simulink model "ASM_Traffic_V2X_Complete_Model_2"  (R2019a)
settings: Solver=ode1  StartTime=SIM.tstart.v  StopTime=Inf  FixedStep=SIM.StepSize.v  RelTol=1e-3
PostLoadFcn:
  | if any(exist('dsrtsu_mdlpostloadfcn', 'file') ~= 0), dsrtsu_mdlpostloadfcn('Execute', bdroot); end
  | try, asm_mdl_postloadfcn(bdroot, 'UpdateModel', 2200); catch, disp(lasterr); end,
undefined symbols (not defined in the file): _SensorPnts_1, _SensorPnts_13, _SensorPnts_17, _SensorPnts_21, _SensorPnts_25, _SensorPnts_29, _SensorPnts_33, _SensorPnts_37, _SensorPnts_41, _SensorPnts_45, _SensorPnts_49, _SensorPnts_5, _SensorPnts_53, _SensorPnts_57, _SensorPnts_9, _to_, CPT, G5A, ITS, MDL, rad, s_to_rpm, SIM
libraries: simulink x169, ASM_VehicleDynamics_lib x126, ASM_Traffic_lib x83, ASM_Utils_lib x49, mdbs x45, ASM_Environment_lib x17, dspindex x12, dsaV2xLibraryAux x10, dsmpblib x6, dsaV2xAsn1Library x4, dsaV2xLibrary x4, ASM_BrakeHydraulics_lib x4
(part 5 of 36)

== system ASM_Traffic_V2X_Complete_Model_2/MDL/SoftECU/Soft_ECU_Engine_Basic ==
  n_Engine[rpm] : Inport
  Trq_Driver_Des[Nm] : Inport  Port=2
  Pos_AccPedal_Driver[%] : Inport  Port=3
  Sw_Ignition[0Off|1On] : Inport  Port=4
  Sw_StarterReq[0Off|1On] : Inport  Port=5
  Reset[] : Inport  Port=6
  Enable_TrqIncrease_Fast_ESP[0|1] : Inport  Port=7
  Trq_IncreaseRequest_Fast_ESP[Nm] : Inport  Port=8
  Enable_TrqDecrease_Fast_ESP[0|1] : Inport  Port=9
  Trq_DecreaseRequest_Fast_ESP[Nm] : Inport  Port=10
  Enable_TrqDecrease_Slow_ESP[0|1] : Inport  Port=11
  Trq_DecreaseRequest_Slow_ESP[Nm] : Inport  Port=12
  Enable_Trq_Extern[0|1] : Inport  Port=13
  Trq_Request_Extern[Nm] : Inport  Port=14
  Factor_Trq_Engine_Red[%] : Inport  Port=15
  ASMSignalCollector : Subsystem
  DisableReset : Subsystem
      mask Display: disp('DisableReset')
  ENGINE_OPERATION_BASIC : ASM_VehicleDynamics_lib/SoftECU/SoftECU_EngineBasic/ENGINE_OPERATION_BASIC  Tag=ASM_SUBCOMPONENT  Const_n_Engine_Min_EngineOn=MDL.SoftECU.EngineBasic.EngineOperation.Const_n_Engine_Min_EngineOn  Const_t_Max_Starter=MDL.SoftECU.EngineBasic.EngineOperation.Const_t_Max_Starter  Const_n_Engine_LowLim_Shutdown=MDL.SoftECU.EngineBasic.EngineOperation.Const_n_Engine_LowLim_Shutdown  Const_t_Shutdown=MDL.SoftECU.EngineBasic.EngineOperation.Const_t_Shutdown  StepSize=SIM.StepSize  ASMProperties=struct('Name','ENGINE_OPERATION_BASIC','Version','1.0','Library','ASM_VehicleDynamics_lib')  ASMInstanceName=engine_operation_basic  ASMInstanceID=1
  IDLE_SPEED_CONTROL_ENGINE_BASIC : ASM_VehicleDynamics_lib/SoftECU/SoftECU_EngineBasic/IDLE_SPEED_CONTROL_ENGINE_BASIC  Tag=ASM_SUBCOMPONENT  Const_n_EngineIdle_Set=MDL.SoftECU.EngineBasic.Const_n_EngineIdle_Set  Const_P_Idle=MDL.SoftECU.EngineBasic.Const_P_Idle  Const_I_Idle=MDL.SoftECU.EngineBasic.Const_I_Idle  StepSize=SIM.StepSize  ASMProperties=struct('Name','IDLE_SPEED_CONTROL_ENGINE_BASIC','Version','4.0','Library','ASM_VehicleDynamics_lib')  ASMInstanceName=idle_speed_control_engine_basic  ASMInstanceID=1
  StarterPermanentOn_Handling : Subsystem
  Sw_n_Engine_Idle_Request[0Off|1On] : Constant  Value=0
  TORQUE_INTERVENTION_FAST_ENGINE_BASIC : ASM_VehicleDynamics_lib/SoftECU/SoftECU_EngineBasic/TORQUE_INTERVENTION_FAST_ENGINE_BASIC  Tag=ASM_SUBCOMPONENT  StepSize=SIM.StepSize  ASMProperties=struct('Name','TORQUE_INTERVENTION_FAST_ENGINE_BASIC','Version','2.0','Library','ASM_VehicleDynamics_lib')  ASMInstanceName=torque_intervention_fast_engine_basic  ASMInstanceID=1
  TORQUE_INTERVENTION_SLOW_ENGINE_BASIC : ASM_VehicleDynamics_lib/SoftECU/SoftECU_EngineBasic/TORQUE_INTERVENTION_SLOW_ENGINE_BASIC  Tag=ASM_SUBCOMPONENT  Map_Trq_Engine_Inv=MDL.SoftECU.EngineBasic.Map_Trq_Engine_Inv  StepSize=SIM.StepSize  ASMProperties=struct('Name','TORQUE_INTERVENTION_SLOW_ENGINE_BASIC','Version','3.0','Library','ASM_VehicleDynamics_lib')  ASMInstanceName=torque_intervention_slow_engine_basic  ASMInstanceID=1
  Torque_Intervention_During_Gear_Shift : Subsystem
  Unit Delay : UnitDelay  SampleTime=-1
  Unit Delay1 : UnitDelay  SampleTime=-1
  n_Engine_Idle_Request[rpm] : Constant  Value=0
  ASMSignalBus : Outport
  Engine_Dynamic_Fast[0|1] : Outport  Port=2
  Pos_AccPedal_Influenced[%] : Outport  Port=3
  Pos_AccPedal_Driver_Des[%] : Outport  Port=4
  Sw_Starter[0Off|1On] : Outport  Port=5
  State_Engine[0|1|2|3|4] : Outport  Port=6
  tag scope: ASMBUS_SoftECU_Engine_EngineOperation=global, ASMBUS_SoftECU_Engine_IdleSpeedControl=global, ASMBUS_SoftECU_Engine_TorqueIntervention_fast=global, ASMBUS_SoftECU_Engine_TorqueIntervention_slow=global
  wires:
  Unit Delay1/1 -> ENGINE_OPERATION_BASIC/2
  Unit Delay/1 -> IDLE_SPEED_CONTROL_ENGINE_BASIC/4, ENGINE_OPERATION_BASIC/1
  StarterPermanentOn_Handling/2(Sw_Starter[0Off|1On]) -> Sw_Starter[0Off|1On]/1
  StarterPermanentOn_Handling/1(ASMSignalBus) -> [ASMBUS_SoftECU_Engine_EngineOperation]
  ENGINE_OPERATION_BASIC/1 -> StarterPermanentOn_Handling/1(ASMSignalBus_)
  Factor_Trq_Engine_Red[%]/1 -> Torque_Intervention_During_Gear_Shift/1(Factor_Trq_Engine_Red[%])
  Torque_Intervention_During_Gear_Shift/1(Pos_AccPedal[%]) -> TORQUE_INTERVENTION_SLOW_ENGINE_BASIC/8
  n_Engine_Idle_Request[rpm]/1 -> IDLE_SPEED_CONTROL_ENGINE_BASIC/7
  Sw_n_Engine_Idle_Request[0Off|1On]/1 -> IDLE_SPEED_CONTROL_ENGINE_BASIC/6
  DisableReset/1(Reset[0|1]) -> ENGINE_OPERATION_BASIC/4
  ENGINE_OPERATION_BASIC/3 -> State_Engine[0|1|2|3|4]/1
  ENGINE_OPERATION_BASIC/2 -> StarterPermanentOn_Handling/2(Sw_Starter[0Off|1On]_)
  Sw_StarterReq[0Off|1On]/1 -> Unit Delay1/1
  ASMSignalCollector/1(ASMSignalBus) -> ASMSignalBus/1
  TORQUE_INTERVENTION_SLOW_ENGINE_BASIC/1 -> [ASMBUS_SoftECU_Engine_TorqueIntervention_slow]
  Trq_DecreaseRequest_Slow_ESP[Nm]/1 -> TORQUE_INTERVENTION_SLOW_ENGINE_BASIC/5
  Enable_TrqDecrease_Slow_ESP[0|1]/1 -> TORQUE_INTERVENTION_SLOW_ENGINE_BASIC/4
  Enable_Trq_Extern[0|1]/1 -> TORQUE_INTERVENTION_SLOW_ENGINE_BASIC/6
  Trq_Request_Extern[Nm]/1 -> TORQUE_INTERVENTION_SLOW_ENGINE_BASIC/7
  Reset[]/1 -> IDLE_SPEED_CONTROL_ENGINE_BASIC/5, DisableReset/1(Reset_VehicleStates[0|1]), TORQUE_INTERVENTION_SLOW_ENGINE_BASIC/3, TORQUE_INTERVENTION_FAST_ENGINE_BASIC/6
  Enable_TrqIncrease_Fast_ESP[0|1]/1 -> TORQUE_INTERVENTION_FAST_ENGINE_BASIC/3
  Trq_IncreaseRequest_Fast_ESP[Nm]/1 -> TORQUE_INTERVENTION_FAST_ENGINE_BASIC/4
  Enable_TrqDecrease_Fast_ESP[0|1]/1 -> TORQUE_INTERVENTION_FAST_ENGINE_BASIC/1
  Trq_DecreaseRequest_Fast_ESP[Nm]/1 -> TORQUE_INTERVENTION_FAST_ENGINE_BASIC/2
  TORQUE_INTERVENTION_FAST_ENGINE_BASIC/1 -> [ASMBUS_SoftECU_Engine_TorqueIntervention_fast]
  IDLE_SPEED_CONTROL_ENGINE_BASIC/1 -> [ASMBUS_SoftECU_Engine_IdleSpeedControl]
  Sw_Ignition[0Off|1On]/1 -> Unit Delay/1
  IDLE_SPEED_CONTROL_ENGINE_BASIC/3 -> Pos_AccPedal_Driver_Des[%]/1
  TORQUE_INTERVENTION_FAST_ENGINE_BASIC/4 -> TORQUE_INTERVENTION_SLOW_ENGINE_BASIC/2
  Pos_AccPedal_Driver[%]/1 -> Torque_Intervention_During_Gear_Shift/2(Pos_AccPedal_Driver[%]), IDLE_SPEED_CONTROL_ENGINE_BASIC/2
  IDLE_SPEED_CONTROL_ENGINE_BASIC/2 -> Pos_AccPedal_Influenced[%]/1
  Trq_Driver_Des[Nm]/1 -> TORQUE_INTERVENTION_FAST_ENGINE_BASIC/5
  TORQUE_INTERVENTION_FAST_ENGINE_BASIC/2 -> Engine_Dynamic_Fast[0|1]/1
  TORQUE_INTERVENTION_SLOW_ENGINE_BASIC/2 -> IDLE_SPEED_CONTROL_ENGINE_BASIC/1
  n_Engine[rpm]/1 -> IDLE_SPEED_CONTROL_ENGINE_BASIC/3, ENGINE_OPERATION_BASIC/3, TORQUE_INTERVENTION_SLOW_ENGINE_BASIC/9
  TORQUE_INTERVENTION_FAST_ENGINE_BASIC/3 -> TORQUE_INTERVENTION_SLOW_ENGINE_BASIC/1

== system ASM_Traffic_V2X_Complete_Model_2/MDL/SoftECU/Soft_ECU_Transmission ==
  n_Engine[rad|s] : Inport  PortDimensions=1
  omega_In_Trm[rad|s] : Inport  Port=2  PortDimensions=1
  omega_Out_Trm[rad|s] : Inport  Port=3
  State_Engine[0|1|2|3|4] : Inport  Port=4
  Gear_Current[] : Inport  Port=5
  Pos_AccPedal_Driver[%] : Inport  Port=6
  SelectorLever[-3T|-2P|-1R|0N|1D] : Inport  Port=7  PortDimensions=1
  TipShift[-1Down|0Off|1Up] : Inport  Port=8
  Gear_Max_Maneuver[0Off|1_n] : Inport  Port=9
  Reset[0|1] : Inport  Port=10
  Gear_Maneuver[] : Inport  Port=11
  GearClutch_Mode[1Stim|2SoftECU|3OpenClutch|4RefGear] : Inport  Port=12
  ASMSignalCollector : Subsystem
  Ctrl_Lockup_Clutch_Maneuver[%] : Constant  Value=0
  Gear_Requested : Sum  SaturateOnIntegerOverflow=on
  Goto Tag Visibility : GotoTagVisibility  GotoTag=ASMBUS_SOFTECU_LOCKUP_CLUTCH_CONTROL
  Goto Tag Visibility1 : GotoTagVisibility  GotoTag=ASMBUS_SOFTECU_SHIFT_STRATEGY
  Goto Tag Visibility2 : GotoTagVisibility  GotoTag=ASMBUS_SOFTECU_TIP_SHIFT_CONTROL
  Goto Tag Visibility3 : GotoTagVisibility  GotoTag=ASMBUS_SOFTECU_TORQUE_INTERVENTION_CONTROL
  Goto Tag Visibility4 : GotoTagVisibility  GotoTag=ASMBUS_SOFTECU_SHIFT_LOCK_CONTROL
  LOCKUP_CLUTCH_CONTROL : ASM_VehicleDynamics_lib/SoftECU/SoftECU_Transmission/LOCKUP_CLUTCH_CONTROL  Tag=ASM_SUBCOMPONENT  Const_P_LockupClutch=MDL.SoftECU.SoftECUTransmission.LockupClutchControl.Const_P_LockupClutch  Const_I_LockupClutch=MDL.SoftECU.SoftECUTransmission.LockupClutchControl.Const_I_LockupClutch  Map_State_LockupClutch=MDL.SoftECU.SoftECUTransmission.LockupClutchControl.Map_State_LockupClutch  StepSize=SIM.StepSize  ASMProperties=struct('Name','LOCKUP_CLUTCH_CONTROL','Version','1.0','Library','ASM_VehicleDynamics_lib')  ASMInstanceName=lockup_clutch_control  ASMInstanceID=1
  SHIFT_LOCK_CONTROL : ASM_VehicleDynamics_lib/SoftECU/SoftECU_Transmission/SHIFT_LOCK_CONTROL  Tag=ASM_SUBCOMPONENT  ASMProperties=struct('Name','SHIFT_LOCK_CONTROL','Version','2.0','Library','ASM_VehicleDynamics_lib')  ASMInstanceName=shift_lock_control  ASMInstanceID=1
  SHIFT_STRATEGY : ASM_VehicleDynamics_lib/SoftECU/SoftECU_Transmission/SHIFT_STRATEGY  Tag=ASM_SUBCOMPONENT  Map_omega_Upshift=MDL.SoftECU.SoftECUTransmission.ShiftStrategy.Map_omega_Upshift  Map_omega_Downshift=MDL.SoftECU.SoftECUTransmission.ShiftStrategy.Map_omega_Downshift  Const_t_Min_Shift=MDL.SoftECU.SoftECUTransmission.ShiftStrategy.Const_t_Min_Shift  StepSize=SIM.StepSize  ASMProperties=struct('Name','SHIFT_STRATEGY','Version','1.0','Library','ASM_VehicleDynamics_lib')  ASMInstanceName=shift_strategy  ASMInstanceID=1
  SOFTECU_SETUP : Subsystem
  Sw_Gear : Subsystem
  Sw_LockupClutch : Subsystem
  TIP_SHIFT_CONTROL : ASM_VehicleDynamics_lib/SoftECU/SoftECU_Transmission/TIP_SHIFT_CONTROL  Tag=ASM_SUBCOMPONENT  ASMProperties=struct('Name','TIP_SHIFT_CONTROL','Version','1.0','Library','ASM_VehicleDynamics_lib')  ASMInstanceName=tip_shift_control  ASMInstanceID=1
  TORQUE_INTERVENTION_CONTROL : ASM_VehicleDynamics_lib/SoftECU/SoftECU_Transmission/TORQUE_INTERVENTION_CONTROL  Tag=ASM_SUBCOMPONENT  Map_Factor_Trq_Engine_Red=MDL.SoftECU.SoftECUTransmission.TorqueInterventionControl.Map_Factor_Trq_Engine_Red  Const_t_Gear_Offs=MDL.SoftECU.SoftECUTransmission.TorqueInterventionControl.Const_t_Gear_Offs  StepSize=SIM.StepSize  ASMProperties=struct('Name','TORQUE_INTERVENTION_CONTROL','Version','1.0','Library','ASM_VehicleDynamics_lib')  ASMInstanceName=torque_intervention_control  ASMInstanceID=1
  Unit Delay : UnitDelay  SampleTime=-1
  Unit Delay1 : UnitDelay  SampleTime=-1
  Unit Delay2 : UnitDelay  InitialCondition=100  SampleTime=-1
      settings: AttributesFormatString=Init = %<InitialCondition>
  UnitConversion1 : ASM_Utils_lib/UnitConversion/UnitConversion  Selection=rad/s_to_rpm
  UnitConversion2 : ASM_Utils_lib/UnitConversion/UnitConversion  Selection=rad/s_to_rpm
  UnitConversion3 : ASM_Utils_lib/UnitConversion/UnitConversion  Selection=rad/s_to_rpm
  ASMSignalBus : Outport
  Factor_Trq_Engine_Red[%] : Outport  Port=2
  Ctrl_Parking_Pawl[0|1] : Outport  Port=3
  Ctrl_Lockup_Clutch[%] : Outport  Port=4
  Gear[] : Outport  Port=5
  tag scope: ASMBUS_SOFTECU_LOCKUP_CLUTCH_CONTROL=scoped, ASMBUS_SOFTECU_SHIFT_LOCK_CONTROL=scoped, ASMBUS_SOFTECU_SHIFT_STRATEGY=scoped, ASMBUS_SOFTECU_TIP_SHIFT_CONTROL=scoped, ASMBUS_SOFTECU_TORQUE_INTERVENTION_CONTROL=scoped
  wires:
  ASMSignalCollector/1(ASMSignalBus) -> ASMSignalBus/1
  TIP_SHIFT_CONTROL/1 -> [ASMBUS_SOFTECU_TIP_SHIFT_CONTROL]
  SHIFT_STRATEGY/1 -> [ASMBUS_SOFTECU_SHIFT_STRATEGY]
  LOCKUP_CLUTCH_CONTROL/1 -> [ASMBUS_SOFTECU_LOCKUP_CLUTCH_CONTROL]
  UnitConversion1/1 -> LOCKUP_CLUTCH_CONTROL/2
  omega_In_Trm[rad|s]/1 -> UnitConversion1/1
  UnitConversion3/1 -> LOCKUP_CLUTCH_CONTROL/1
  n_Engine[rad|s]/1 -> UnitConversion3/1
  Ctrl_Lockup_Clutch_Maneuver[%]/1 -> LOCKUP_CLUTCH_CONTROL/3
  TipShift[-1Down|0Off|1Up]/1 -> TIP_SHIFT_CONTROL/3
  Gear_Current[]/1 -> TIP_SHIFT_CONTROL/2
  omega_Out_Trm[rad|s]/1 -> UnitConversion2/1
  Gear_Maneuver[]/1 -> SHIFT_STRATEGY/3
  GearClutch_Mode[1Stim|2SoftECU|3OpenClutch|4RefGear]/1 -> Sw_LockupClutch/1(In[]), Sw_Gear/1(In[])
  SelectorLever[-3T|-2P|-1R|0N|1D]/1 -> SHIFT_LOCK_CONTROL/1, TIP_SHIFT_CONTROL/1, SHIFT_STRATEGY/1
  Gear_Max_Maneuver[0Off|1_n]/1 -> SOFTECU_SETUP/1(Gear_Max_Maneuver[0Off|1_n])
  Unit Delay2/1 -> Ctrl_Lockup_Clutch[%]/1
  Unit Delay1/1 -> Gear[]/1
  Unit Delay/1 -> Ctrl_Parking_Pawl[0|1]/1
  SHIFT_LOCK_CONTROL/2 -> Unit Delay/1
  LOCKUP_CLUTCH_CONTROL/2 -> Unit Delay2/1
  TIP_SHIFT_CONTROL/2 -> Gear_Requested/2
  SHIFT_STRATEGY/2 -> Gear_Requested/1
  Gear_Requested/1 -> TORQUE_INTERVENTION_CONTROL/1
  UnitConversion2/1 -> SHIFT_STRATEGY/2, LOCKUP_CLUTCH_CONTROL/4
  State_Engine[0|1|2|3|4]/1 -> TIP_SHIFT_CONTROL/4, SHIFT_STRATEGY/6
  Reset[0|1]/1 -> LOCKUP_CLUTCH_CONTROL/7, SHIFT_LOCK_CONTROL/2, SHIFT_STRATEGY/7, TIP_SHIFT_CONTROL/5, TORQUE_INTERVENTION_CONTROL/2
  Sw_LockupClutch/1(Sw_LockupClutch[]) -> LOCKUP_CLUTCH_CONTROL/5
  Sw_Gear/1(Sw_Gear[]) -> SHIFT_STRATEGY/4
  SHIFT_LOCK_CONTROL/1 -> [ASMBUS_SOFTECU_SHIFT_LOCK_CONTROL]
  Pos_AccPedal_Driver[%]/1 -> LOCKUP_CLUTCH_CONTROL/6, SHIFT_STRATEGY/5
  TORQUE_INTERVENTION_CONTROL/1 -> [ASMBUS_SOFTECU_TORQUE_INTERVENTION_CONTROL]
  TORQUE_INTERVENTION_CONTROL/3 -> Unit Delay1/1
  TORQUE_INTERVENTION_CONTROL/2 -> Factor_Trq_Engine_Red[%]/1

== system ASM_Traffic_V2X_Complete_Model_2/MDL/SoftECU/StarterPermanentOn_Handling ==
  Bus Selector : BusSelector  OutputSignals=Sw_Starter_Mode[1Stim|2PermanentOn]
  PowerOff : Constant  Value=-1
  SoftECU : Constant  Value=2
  StarterOn : Constant  Value=2
  StarterPermanantOn : simulink/Logic and Bit Operations/Compare To Constant  relop===  const=2  OutDataTypeStr=boolean
  Stim : Constant
  Switch : Switch  Criteria=u2 ~= 0
  Switch1 : Switch  Criteria=u2 ~= 0
  State_StartButton_Ext[-1|0|1|2] : Outport
  Mode_StartButtonState[1Stim|2SoftECU] : Outport  Port=2
  wires:
  StarterPermanantOn/1 -> Switch1/2, Switch/2
  Switch1/1 -> State_StartButton_Ext[-1|0|1|2]/1
  Bus Selector/1 -> StarterPermanantOn/1  "<Sw_Starter_Mode[1Stim|2PermanentOn]>"
  Stim/1 -> Switch/1
  [TAG_StartButton_Signals] -> Bus Selector/1
  Switch/1 -> Mode_StartButtonState[1Stim|2SoftECU]/1
  SoftECU/1 -> Switch/3
  StarterOn/1 -> Switch1/1
  PowerOff/1 -> Switch1/3

== system ASM_Traffic_V2X_Complete_Model_2/MDL/VehicleDynamics/ASMSignalCollector ==
  BusCreator : BusCreator  Inputs=7
  tag scope: ASMBUS_VehicleDynamics=global
  wires:
  [ASMBUS_VehicleDynamics_Suspension] -> BusCreator/7
  BusCreator/1 -> [ASMBUS_VehicleDynamics]  "VehicleDynamics"
  [ASMBUS_VehicleDynamics_Brake] -> BusCreator/6
  [ASMBUS_VehicleDynamics_Steering] -> BusCreator/5
  [ASMBUS_VehicleDynamics_WheelSpeed] -> BusCreator/4
  [ASMBUS_VehicleDynamics_Aerodynamics] -> BusCreator/3
  [ASMBUS_VehicleDynamics_Tire] -> BusCreator/2
  [ASMBUS_VehicleDynamics_VehicleMovement] -> BusCreator/1

== system ASM_Traffic_V2X_Complete_Model_2/MDL/VehicleDynamics/Brake ==
  Reset[] : Inport
  Pos_BrakePedal[%] : Inport  Port=2
  IO_Signals : Inport  Port=3
  p_Ambient[Pa] : Inport  Port=4
  Sw_ParkingBrake[0Off|1On] : Inport  Port=5
  T_Ambient[degC] : Inport  Port=6
  Pos_AccPedal[%] : Inport  Port=7
  ASMSignalCollector : Subsystem
  BRAKE_BOOSTER : ASM_VehicleDynamics_lib/VehicleDynamics/Brake/BRAKE_BOOSTER  Tag=ASM_SUBCOMPONENT  Const_F_OutputPoint=MDL.VehicleDynamics.BrakeBooster.Const_F_OutputPoint  Const_p_OutputPoint=MDL.VehicleDynamics.BrakeBooster.Const_p_OutputPoint  Const_F_Max_PistonRod=MDL.VehicleDynamics.BrakeBooster.Const_F_Max_PistonRod  Const_p_nom_VaccumChamber=MDL.VehicleDynamics.BrakeBooster.Const_p_nom_VaccumChamber  Const_V_VacuumChamber=MDL.VehicleDynamics.BrakeBooster.Const_V_VacuumChamber  Const_V_RearChamber=MDL.VehicleDynamics.BrakeBooster.Const_V_RearChamber  Const_A_Connect_BellValve=MDL.VehicleDynamics.BrakeBooster.Const_A_Connect_BellValve  Const_A_Boost_BellValve=MDL.VehicleDynamics.BrakeBooster.Const_A_Boost_BellValve  Const_A_MainfoldValve=MDL.VehicleDynamics.BrakeBooster.Const_A_MainfoldValve  Const_A_Leakage_MainfoldValve=MDL.VehicleDynamics.BrakeBooster.Const_A_Leakage_MainfoldValve  Const_c_spring=MDL.VehicleDynamics.BrakeBooster.Const_c_spring  StepSize=SIM.StepSize  ASMProperties=struct('Name','BRAKE_BOOSTER','Version','2.0','Library','ASM_VehicleDynamics_lib')  ASMInstanceName=BrakeBooster  ASMInstanceID=1
  BRAKE_DISC : ASM_VehicleDynamics_lib/VehicleDynamics/Brake/BRAKE_DISC  Tag=ASM_SUBCOMPONENT  Const_Fric_Coef_FL=MDL.VehicleDynamics.BrakeDisc.FL.Const_Coef_Fric  Const_Fric_Coef_FR=MDL.VehicleDynamics.BrakeDisc.FR.Const_Coef_Fric  Const_Fric_Coef_RL=MDL.VehicleDynamics.BrakeDisc.RL.Const_Coef_Fric  Const_Fric_Coef_RR=MDL.VehicleDynamics.BrakeDisc.RR.Const_Coef_Fric  Const_A_FL=MDL.VehicleDynamics.BrakeDisc.FL.Const_A_Fric  Const_A_FR=MDL.VehicleDynamics.BrakeDisc.FR.Const_A_Fric  Const_A_RL=MDL.VehicleDynamics.BrakeDisc.RL.Const_A_Fric  Const_A_RR=MDL.VehicleDynamics.BrakeDisc.RR.Const_A_Fric  Const_r_FL=MDL.VehicleDynamics.BrakeDisc.FL.Const_r  Const_r_FR=MDL.VehicleDynamics.BrakeDisc.FR.Const_r  Const_r_RL=MDL.VehicleDynamics.BrakeDisc.RL.Const_r  Const_r_RR=MDL.VehicleDynamics.BrakeDisc.RR.Const_r  ASMProperties=struct('Name','BRAKE_DISC','Version','4.0','Library','ASM_VehicleDynamics_lib')  ASMInstanceName=brake_disc  ASMInstanceID=1
  BRAKE_HYDRAULICS : Subsystem  Tag=ASM_BRAKE_HYDRAULICS
      settings: CopyFcn=asm_blk_copy_gui('start','usecase','brakehydraulicscopy')
  Bus Selector : BusSelector  OutputSignals=Valves.Ctrl_HydPump[0_1],Valves.Ctrl_PreChargeValve_1[0_1],Valves.Ctrl_PreChargeValve_2[0_1],Valves.Ctrl_ChangeOverValve_1[0_1],Valves.Ctrl_ChangeOverValve_2[0_1],Valves.Ctrl_InletValve_FL[0_1],Valves.Ctrl_InletValve_FR[0_1],Valves.Ctrl_InletValve_RL[0_1],Valves.Ctrl_InletValve_RR[0_1],Valves.Ctrl_OutletValve_FL[0_1],Valves.Ctrl_OutletValve_FR[0_1],Valves.Ctrl_OutletValve_RL[0_1],Valves.Ctrl_OutletValve_RR[0_1],ECU_Mode.ECU_ESP_Mode[0None|1ABS|2ESP|3ASR]
  Bus Selector1 : BusSelector  OutputSignals=DesiredPressure.Enable_p_Brake_Desired[0|1],DesiredPressure.p_Brake_Desired[bar]
  Constant : Constant  Value=0
  ForceParkingBrake : Subsystem
  MANIFOLD_PRESSURE : ASM_VehicleDynamics_lib/VehicleDynamics/Brake/MANIFOLD_PRESSURE  Tag=ASM_SUBCOMPONENT  Map_p_Man=MDL.VehicleDynamics.Manifold.Map_p_Man  ASMProperties=struct('Name','MANIFOLD_PRESSURE','Version','2.0','Library','ASM_VehicleDynamics_lib')  ASMInstanceName=BrakeBooster  ASMInstanceID=1
  MASTER_BRAKE_CYLINDER : ASM_BrakeHydraulics_lib/BrakeHydraulics/BrakeCylinders/MASTER_BRAKE_CYLINDER  Tag=ASM_SUBCOMPONENT  Const_p_max=MDL.BrkHyd.MasterBrakeCylinderLinear.Const_p_max  Map_BrakeForce=MDL.BrkHyd.MasterBrakeCylinder.Map_BrakeForce  Const_r_piston=MDL.BrkHyd.MasterBrakeCylinder.Const_r_piston  Const_displ_max_piston=MDL.BrkHyd.MasterBrakeCylinder.Const_displ_max_piston  ASMProperties=struct('Name','MASTER_BRAKE_CYLINDER','Version','7.0','Library','ASM_BrakeHydraulics_lib')  ASMInstanceName=MasterBrakeCylinder  ASMInstanceID=1
  OpenBrkHydModel : Subsystem
      settings: OpenFcn=asm_open_lib('ASM_BrakeHydraulics_lib/Demos');
      mask Display: disp('Open\nASM_Brakehydraulics_lib')
  UnitConversion : ASM_Utils_lib/UnitConversion/UnitConversion  Selection=Pa_to_bar
  ASMSignalBus : Outport
  Trq_Brake[FL,FR,RL,RR][Nm] : Outport  Port=2
  tag scope: ASMBUS_VehicleDynamics_BrakeBooster=global, ASMBUS_VehicleDynamics_BrakeDisc=global, ASMBUS_VehicleDynamics_BrakeHydraulics=global, ASMBUS_VehicleDynamics_Manifold=global, TAG_DISP_BrkHyd_MasterBrakeCylinder=global
  wires:
  BRAKE_HYDRAULICS/2(p_Brake[FL,FR,RL,RR][bar]) -> BRAKE_DISC/1
  ForceParkingBrake/1(F_ParkingBrake[FL;FR;RL;RR][N]) -> BRAKE_DISC/4
  MANIFOLD_PRESSURE/2 -> BRAKE_BOOSTER/7
  T_Ambient[degC]/1 -> BRAKE_BOOSTER/4, BRAKE_BOOSTER/6
  Constant/1 -> BRAKE_BOOSTER/5
  Pos_AccPedal[%]/1 -> MANIFOLD_PRESSURE/1
  p_Ambient[Pa]/1 -> UnitConversion/1
  UnitConversion/1 -> MASTER_BRAKE_CYLINDER/3, BRAKE_HYDRAULICS/18(p_Ambient[bar]), BRAKE_DISC/3, BRAKE_BOOSTER/3
  MANIFOLD_PRESSURE/1 -> [ASMBUS_VehicleDynamics_Manifold]
  BRAKE_BOOSTER/1 -> [ASMBUS_VehicleDynamics_BrakeBooster]
  Sw_ParkingBrake[0Off|1On]/1 -> ForceParkingBrake/1(Sw_ParkingBrake[0Off|1On])
  Bus Selector/13 -> BRAKE_HYDRAULICS/16(Ctrl_OutletValve_RR[])  "<Ctrl_OutletValve_RR[0_1]>"
  Bus Selector/12 -> BRAKE_HYDRAULICS/15(Ctrl_OutletValve_RL[])  "<Ctrl_OutletValve_RL[0_1]>"
  Bus Selector/11 -> BRAKE_HYDRAULICS/14(Ctrl_OutletValve_FR[])  "<Ctrl_OutletValve_FR[0_1]>"
  Bus Selector/10 -> BRAKE_HYDRAULICS/13(Ctrl_OutletValve_FL[])  "<Ctrl_OutletValve_FL[0_1]>"
  Bus Selector/9 -> BRAKE_HYDRAULICS/12(Ctrl_InletValve_RR[])  "<Ctrl_InletValve_RR[0_1]>"
  Bus Selector/8 -> BRAKE_HYDRAULICS/11(Ctrl_InletValve_RL[])  "<Ctrl_InletValve_RL[0_1]>"
  Bus Selector/7 -> BRAKE_HYDRAULICS/10(Ctrl_InletValve_FR[])  "<Ctrl_InletValve_FR[0_1]>"
  Bus Selector/6 -> BRAKE_HYDRAULICS/9(Ctrl_InletValve_FL[])  "<Ctrl_InletValve_FL[0_1]>"
  Bus Selector/5 -> BRAKE_HYDRAULICS/8(Ctrl_ChangeOverValve_2[])  "<Ctrl_ChangeOverValve_2[0_1]>"
  Bus Selector/4 -> BRAKE_HYDRAULICS/7(Ctrl_ChangeOverValve_1[])  "<Ctrl_ChangeOverValve_1[0_1]>"
  Bus Selector/3 -> BRAKE_HYDRAULICS/6(Ctrl_PreChargeValve_2[])  "<Ctrl_PreChargeValve_2[0_1]>"
  Bus Selector/2 -> BRAKE_HYDRAULICS/5(Ctrl_PreChargeValve_1[])  "<Ctrl_PreChargeValve_1[0_1]>"
  Bus Selector/1 -> BRAKE_HYDRAULICS/4(Ctrl_HydPump[0_1])  "<Ctrl_HydPump[0_1]>"
  Pos_BrakePedal[%]/1 -> BRAKE_BOOSTER/8, MASTER_BRAKE_CYLINDER/1
  Reset[]/1 -> BRAKE_BOOSTER/9, BRAKE_HYDRAULICS/3(Reset[])
  BRAKE_HYDRAULICS/1(ASMSignalBus) -> [ASMBUS_VehicleDynamics_BrakeHydraulics]
  IO_Signals/1 -> Bus Selector/1, Bus Selector1/1
  BRAKE_DISC/1 -> [ASMBUS_VehicleDynamics_BrakeDisc]
  BRAKE_DISC/2 -> Trq_Brake[FL,FR,RL,RR][Nm]/1
  ASMSignalCollector/1(ASMSignalBus) -> ASMSignalBus/1
  Bus Selector/14 -> BRAKE_HYDRAULICS/17(ECU_Mode[0None|1ABS|2ESP|3ASR])  "<ECU_ESP_Mode[0None|1ABS|2ESP|3ASR]>"
  [TAG_Sw_DistributionPattern] -> BRAKE_HYDRAULICS/2(Sw_DistributionPattern[1X|2II])
  MASTER_BRAKE_CYLINDER/3 -> BRAKE_HYDRAULICS/1(p_MasterBrakeCylinder[bar]), BRAKE_BOOSTER/1
  MASTER_BRAKE_CYLINDER/4 -> BRAKE_BOOSTER/2
  MASTER_BRAKE_CYLINDER/2 -> BRAKE_DISC/2
  Bus Selector1/1 -> MASTER_BRAKE_CYLINDER/5  "<Enable_p_Brake_Desired[0|1]>"
  Bus Selector1/2 -> MASTER_BRAKE_CYLINDER/6  "<p_Brake_Desired[bar]>"
  BRAKE_BOOSTER/2 -> MASTER_BRAKE_CYLINDER/4
  MASTER_BRAKE_CYLINDER/1 -> [TAG_DISP_BrkHyd_MasterBrakeCylinder]
  [TAG_Sw_MasterBrakeCylinder_Mode] -> MASTER_BRAKE_CYLINDER/2

== system ASM_Traffic_V2X_Complete_Model_2/MDL/VehicleDynamics/CommonVehicleParameters ==
  Bus Selector : BusSelector  OutputSignals=Front.Const_m_Left_Wheel[kg],Front.Const_m_Right_Wheel[kg],Rear.Const_m_Left_Wheel[kg],Rear.Const_m_Right_Wheel[kg],Front.Const_Inertia_Tensor_Left_Wheel[3x3][kgm2],Front.Const_Inertia_Tensor_Right_Wheel[3x3][kgm2],Rear.Const_Inertia_Tensor_Left_Wheel[3x3][kgm2],Rear.Const_Inertia_Tensor_Right_Wheel[3x3][kgm2],Front.Const_Inertia_y_Left_Wheel[kgm2],Front.Const_Inertia_y_Right_Wheel[kgm2],Rear.Const_Inertia_y_Left_Wheel[kgm2],Rear.Const_Inertia_y_Right_Wheel[kgm2],Front.Const_Coef_DynamicBrakeTrq_Left_Wheel[Nm|(rad|s)],Front.Const_Coef_DynamicBrakeTrq_Right_Wheel[Nm|(rad|s)],Rear.Const_Coef_DynamicBrakeTrq_Left_Wheel[Nm|(rad|s)],Rear.Const_Coef_DynamicBrakeTrq_Right_Wheel[Nm|(rad|s)]
  COMMON_VEHICLE_PARAMETERS : ASM_VehicleDynamics_lib/VehicleDynamics/Common_Parameter/COMMON_VEHICLE_PARAMETERS  Tag=ASM_SUBCOMPONENT  Const_m_FL_Wheel=MDL.VehicleDynamics.Wheel.FL.Const_m  Const_m_FR_Wheel=MDL.VehicleDynamics.Wheel.FR.Const_m  Const_m_RL_Wheel=MDL.VehicleDynamics.Wheel.RL.Const_m  Const_m_RR_Wheel=MDL.VehicleDynamics.Wheel.RR.Const_m  Const_Inertia_Tensor_FL_Wheel=MDL.VehicleDynamics.Wheel.FL.Const_Inertia_Tensor  Const_Inertia_Tensor_FR_Wheel=MDL.VehicleDynamics.Wheel.FR.Const_Inertia_Tensor  Const_Inertia_Tensor_RL_Wheel=MDL.VehicleDynamics.Wheel.RL.Const_Inertia_Tensor  Const_Inertia_Tensor_RR_Wheel=MDL.VehicleDynamics.Wheel.RR.Const_Inertia_Tensor  Const_Inertia_y_FL_Wheel=MDL.VehicleDynamics.Wheel.FL.Const_Inertia_y  Const_Inertia_y_FR_Wheel=MDL.VehicleDynamics.Wheel.FR.Const_Inertia_y  Const_Inertia_y_RL_Wheel=MDL.VehicleDynamics.Wheel.RL.Const_Inertia_y  Const_Inertia_y_RR_Wheel=MDL.VehicleDynamics.Wheel.RR.Const_Inertia_y  Const_Coef_DynamicBrakeTrq_FL=MDL.VehicleDynamics.Wheel.FL.Const_Coef_DynamicBrakeTrq  Const_Coef_DynamicBrakeTrq_FR=MDL.VehicleDynamics.Wheel.FR.Const_Coef_DynamicBrakeTrq  Const_Coef_DynamicBrakeTrq_RL=MDL.VehicleDynamics.Wheel.RL.Const_Coef_DynamicBrakeTrq  Const_Coef_DynamicBrakeTrq_RR=MDL.VehicleDynamics.Wheel.RR.Const_Coef_DynamicBrakeTrq  ASMProperties=struct('Name','COMMON_VEHICLE_PARAMETERS','Version','3.0','Library','ASM_VehicleDynamics_lib')  ASMInstanceName=common_vehicle_parameters  ASMInstanceID=1
  Mux : Mux
  Mux2 : Mux
  Rename1 : Subsystem
      mask Display: disp('')
  Rename2 : Subsystem
      mask Display: disp('')
  Rename3 : Subsystem
      mask Display: disp('')
  Rename4 : Subsystem
      mask Display: disp('')
  Rename5 : Subsystem
      mask Display: disp('')
  Rename6 : Subsystem
      mask Display: disp('')
  Rename7 : Subsystem
      mask Display: disp('')
  Rename8 : Subsystem
      mask Display: disp('')
  tag scope: TAG_VehicleDynamics_Coef_DynamicBrakeTrq=global, TAG_VehicleDynamics_Inertia_FL_Wheel=global, TAG_VehicleDynamics_Inertia_FR_Wheel=global, TAG_VehicleDynamics_Inertia_RL_Wheel=global, TAG_VehicleDynamics_Inertia_RR_Wheel=global, TAG_VehicleDynamics_Inertia_y_FL_Wheel=global, TAG_VehicleDynamics_Inertia_y_FR_Wheel=global, TAG_VehicleDynamics_Inertia_y_RL_Wheel=global, TAG_VehicleDynamics_Inertia_y_RR_Wheel=global, TAG_VehicleDynamics_Inertia_y_Wheel=global, TAG_VehicleDynamics_m_FL_Wheel=global, TAG_VehicleDynamics_m_FR_Wheel=global, TAG_VehicleDynamics_m_RL_Wheel=global, TAG_VehicleDynamics_m_RR_Wheel=global
  wires:
  Mux/1 -> [TAG_VehicleDynamics_Coef_DynamicBrakeTrq]
  COMMON_VEHICLE_PARAMETERS/1 -> Bus Selector/1
  Bus Selector/1 -> [TAG_VehicleDynamics_m_FL_Wheel]  "<Const_m_Left_Wheel[kg]>"
  Bus Selector/2 -> [TAG_VehicleDynamics_m_FR_Wheel]  "<Const_m_Right_Wheel[kg]>"
  Bus Selector/3 -> [TAG_VehicleDynamics_m_RL_Wheel]  "<Const_m_Left_Wheel[kg]>"
  Bus Selector/4 -> [TAG_VehicleDynamics_m_RR_Wheel]  "<Const_m_Right_Wheel[kg]>"
  Bus Selector/5 -> [TAG_VehicleDynamics_Inertia_FL_Wheel]  "<Const_Inertia_Tensor_Left_Wheel[3x3][kgm2]>"
  Bus Selector/6 -> [TAG_VehicleDynamics_Inertia_FR_Wheel]  "<Const_Inertia_Tensor_Right_Wheel[3x3][kgm2]>"
  Bus Selector/7 -> [TAG_VehicleDynamics_Inertia_RL_Wheel]  "<Const_Inertia_Tensor_Left_Wheel[3x3][kgm2]>"
  Bus Selector/8 -> [TAG_VehicleDynamics_Inertia_RR_Wheel]  "<Const_Inertia_Tensor_Right_Wheel[3x3][kgm2]>"
  Bus Selector/9 -> [TAG_VehicleDynamics_Inertia_y_FL_Wheel], Rename8/1(In1)  "<Const_Inertia_y_Left_Wheel[kgm2]>"
  Bus Selector/10 -> [TAG_VehicleDynamics_Inertia_y_FR_Wheel], Rename5/1(In1)  "<Const_Inertia_y_Right_Wheel[kgm2]>"
  Bus Selector/11 -> [TAG_VehicleDynamics_Inertia_y_RL_Wheel], Rename6/1(In1)  "<Const_Inertia_y_Left_Wheel[kgm2]>"
  Bus Selector/12 -> [TAG_VehicleDynamics_Inertia_y_RR_Wheel], Rename7/1(In1)  "<Const_Inertia_y_Right_Wheel[kgm2]>"
  Bus Selector/13 -> Rename4/1(In1)  "<Const_Coef_DynamicBrakeTrq_Left_Wheel[Nm|(rad|s)]>"
  Bus Selector/14 -> Rename1/1(In1)  "<Const_Coef_DynamicBrakeTrq_Right_Wheel[Nm|(rad|s)]>"
  Bus Selector/15 -> Rename2/1(In1)  "<Const_Coef_DynamicBrakeTrq_Left_Wheel[Nm|(rad|s)]>"
  Bus Selector/16 -> Rename3/1(In1)  "<Const_Coef_DynamicBrakeTrq_Right_Wheel[Nm|(rad|s)]>"
  Rename4/1(Out1) -> Mux/1
  Rename1/1(Out1) -> Mux/2
  Rename2/1(Out1) -> Mux/3
  Rename3/1(Out1) -> Mux/4
  Rename8/1(Out1) -> Mux2/1
  Rename5/1(Out1) -> Mux2/2
  Rename6/1(Out1) -> Mux2/3
  Rename7/1(Out1) -> Mux2/4
  Mux2/1 -> [TAG_VehicleDynamics_Inertia_y_Wheel]

== system ASM_Traffic_V2X_Complete_Model_2/MDL/VehicleDynamics/DerivativeAddition ==
  Angle_SteeringWheel_Driver[deg] : Inport
  Discrete Derivative : simulink/Discrete/Discrete Derivative  gainval=1.0  ICPrevScaledInput=0.0  OutMin=[]  OutMax=[]  OutDataType=fixdt(1, 16)  OutScaling=2^-10  DoSatur=off
  Mux : Mux  Inputs=2
  SteeringWheel_Driver[Angle;Angle_dt][deg;deg|s] : Outport
  wires:
  Angle_SteeringWheel_Driver[deg]/1 -> Discrete Derivative/1, Mux/1
  Mux/1 -> SteeringWheel_Driver[Angle;Angle_dt][deg;deg|s]/1
  Discrete Derivative/1 -> Mux/2

== system ASM_Traffic_V2X_Complete_Model_2/MDL/VehicleDynamics/OR ==
  In1 : Inport
  In2 : Inport  Port=2
  Data Type Conversion : DataTypeConversion  OutDataTypeStr=double
  Logical Operator : Logic  Operator=OR  AllPortsSameDT=off
  Out : Outport
  wires:
  Data Type Conversion/1 -> Out/1
  In2/1 -> Logical Operator/2
  In1/1 -> Logical Operator/1
  Logical Operator/1 -> Data Type Conversion/1

== system ASM_Traffic_V2X_Complete_Model_2/MDL/VehicleDynamics/Suspension ==
  q_Wheel[q1_Front;q2_Front;q1_Rear;q2_Rear][] : Inport  PortDimensions=4
  q_Wheel_dt[q1_Front;q2_Front;q1_Rear;q2_Rear][] : Inport  Port=2  PortDimensions=4
  F_Tire[FL;FR;RL;RR][x;y;z][N] : Inport  Port=3
  Trq_Tire[FL;FR;RL;RR][x;y;z][N|m] : Inport  Port=4
  AirSuspensionSignals_In : Inport  Port=5
  Reset[] : Inport  Port=6
  ASMSignalCollector : Subsystem
  Constant : Constant  Value=0
  Mux{1,5..7,15} (5 alike) : Mux  Inputs=2
  SuspensionFront : Subsystem
  SuspensionRear : Subsystem
  Terminator : Terminator
  Terminator1 : Terminator
  ASMSignalBus : Outport
  SuspensionKinematicRelations_Front : Outport  Port=2
  SuspensionKinematicRelations_Rear : Outport  Port=3
  gFront_dq_Front_dt[2x2][] : Outport  Port=4
  gRear_dq_Rear_dt[2x2][] : Outport  Port=5
  v_Rel_WheelBody[FL,FR,RL,RR][x;y;z][m|s] : Outport  Port=6
  w_Rel_WheelBody[FL,FR,RL,RR][x;y;z][x;y;z][rad|s] : Outport  Port=7
  Pos_Wheels[FL,FR,RL,RR][x;y;z][m] : Outport  Port=8
  gF_Susp[q1_Front;q2_Front;q1_Rear;q2_Rear][] : Outport  Port=9
  UnitVec_y_Wheel_CoorSys_V[FL,FR,RL,RR][x;y;z] : Outport  Port=10
  AirSuspensionSignals_Out : Outport  Port=11
  wires:
  SuspensionRear/8(AirSuspensionSignals_Rear) -> Terminator1/1
  SuspensionFront/8(AirSuspensionSignals_Front) -> Terminator/1
  AirSuspensionSignals_In/1 -> SuspensionFront/5(AirSuspensionSignals_In), SuspensionRear/5(AirSuspensionSignals_In)
  Constant/1 -> AirSuspensionSignals_Out/1
  Reset[]/1 -> SuspensionFront/6(Reset[]), SuspensionRear/6(Reset[])
  q_Wheel[q1_Front;q2_Front;q1_Rear;q2_Rear][]/1 -> SuspensionFront/2(q_Wheel[q1_Front;q2_Front;q1_Rear;q2_Rear][]), SuspensionRear/2(q_Wheel[q1_Front;q2_Front;q1_Rear;q2_Rear][])
  Mux1/1 -> gF_Susp[q1_Front;q2_Front;q1_Rear;q2_Rear][]/1
  SuspensionRear/7(SuspensionKinematicRelations_Rear) -> SuspensionKinematicRelations_Rear/1
  SuspensionFront/7(SuspensionKinematicRelations_Front) -> SuspensionKinematicRelations_Front/1
  SuspensionRear/6(gRear_dq_Rear_dt[2x2][]) -> gRear_dq_Rear_dt[2x2][]/1
  SuspensionFront/6(gFront_dq_Front_dt[2x2][]) -> gFront_dq_Front_dt[2x2][]/1
  SuspensionRear/4(w_Rel_WheelBody[RL,RR][x;y;z][rad|s]) -> Mux7/2
  SuspensionRear/3(v_Rel_WheelBody[RL;RR][x;y;z][m|s]) -> Mux5/2
  SuspensionRear/2(UnitVec_y_Wheel_CoorSys_V[RL;RR][x;y;z][]) -> Mux15/2
  SuspensionRear/5(gF_Rear_Susp[q1,q2][]) -> Mux1/2
  SuspensionFront/5(gF_Front_Susp[q1,q2][]) -> Mux1/1
  SuspensionFront/4(w_Rel_WheelBody[FL,FR][x;y;z][rad|s]) -> Mux7/1
  SuspensionFront/3(v_Rel_WheelBody[FL,FR][x;y;z][m|s]) -> Mux5/1
  SuspensionFront/2(UnitVec_y_Wheel_CoorSys_V[FL,FR][x;y;z]) -> Mux15/1
  SuspensionRear/1("Pos_Wheel[RL;RR][x;y;z][m] ") -> Mux6/2
  Mux15/1 -> UnitVec_y_Wheel_CoorSys_V[FL,FR,RL,RR][x;y;z]/1
  Mux6/1 -> Pos_Wheels[FL,FR,RL,RR][x;y;z][m]/1
  SuspensionFront/1("Pos_Wheel[FL,FR][x;y;z][m] ") -> Mux6/1
  F_Tire[FL;FR;RL;RR][x;y;z][N]/1 -> SuspensionFront/3(F_Tire[FL;FR;RL;RR][x;y;z][N]), SuspensionRear/3(F_Tire[FL;FR;RL;RR][x;y;z][N])
  Mux7/1 -> w_Rel_WheelBody[FL,FR,RL,RR][x;y;z][x;y;z][rad|s]/1
  Mux5/1 -> v_Rel_WheelBody[FL,FR,RL,RR][x;y;z][m|s]/1
  Trq_Tire[FL;FR;RL;RR][x;y;z][N|m]/1 -> SuspensionFront/4(Trq_Tire[FL;FR;RL;RR][x;y;z][N|m]), SuspensionRear/4(Trq_Tire[FL;FR;RL;RR][x;y;z][N|m])
  q_Wheel_dt[q1_Front;q2_Front;q1_Rear;q2_Rear][]/1 -> SuspensionFront/1(q_Wheel_dt[q1_Front;q2_Front;q1_Rear;q2_Rear][]), SuspensionRear/1(q_Wheel_dt[q1_Front;q2_Front;q1_Rear;q2_Rear][])
  ASMSignalCollector/1(ASMSignalBus) -> ASMSignalBus/1

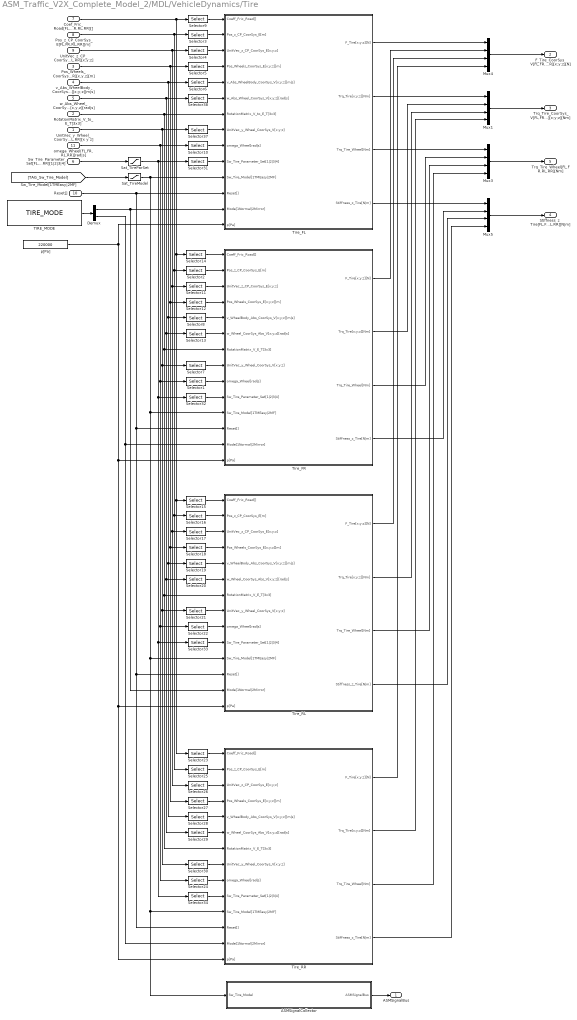
== system ASM_Traffic_V2X_Complete_Model_2/MDL/VehicleDynamics/Tire ==
  UnitVec_y_Wheel_CoorSys_V[FL,FR,RL,RR][x y z] : Inport
  RotationMatrix_V_to_E_T[3x3] : Inport  Port=2
  Pos_Wheels_CoorSys_E[FL,FR,RL,RR][x,y,z][m] : Inport  Port=3
  v_Abs_WheelBody_CoorSys_V[FL,FR,RL,RR][x;y;z][m|s] : Inport  Port=4
  w_Abs_Wheel_CoorSys_V[FL,FR,RL,RR][x,y,z][rad|s] : Inport  Port=5
  Sw_Tire_Parameter_Set[FL,FR,RL,RR][1|2|3|4] : Inport  Port=6
  Coef_Fric_Road[FL,FR,RL,RR][] : Inport  Port=7
  " Pos_z_CP_CoorSys_E[FL,FR,RL,RR][m]" : Inport  Port=8
  UnitVec_z_CP_CoorSys_E[FL,FR,RL,RR][x;y;z] : Inport  Port=9
  Reset[] : Inport  Port=10
  omega_Wheel[FL,FR,RL,RR][rad|s] : Inport  Port=11
  ASMSignalCollector : Subsystem
  Demux : Demux  Outputs=[1 1]
  Mux{1,3..5} (4 alike) : Mux
  Sat_TireModel : Saturate  UpperLimit=2  LowerLimit=1
  Sat_TireParSet : Saturate  UpperLimit=4  LowerLimit=1
  Selector{1..2,14,32} (4 alike) : Selector  InputPortWidth=4  IndexOptions=Index vector (dialog)  Indices=[2]  OutputSizes=1
  Selector{3,9..10,31} (4 alike) : Selector  InputPortWidth=4  IndexOptions=Index vector (dialog)  Indices=[1]  OutputSizes=1
  Selector{7..8,11..13} (5 alike) : Selector  InputPortWidth=12  IndexOptions=Index vector (dialog)  Indices=[4 5 6]  OutputSizes=1
  Selector{15..16,22,33} (4 alike) : Selector  InputPortWidth=4  IndexOptions=Index vector (dialog)  Indices=[3]  OutputSizes=1
  Selector{17..21} (5 alike) : Selector  InputPortWidth=12  IndexOptions=Index vector (dialog)  Indices=[7 8 9]  OutputSizes=1
  Selector{23..25,34} (4 alike) : Selector  InputPortWidth=4  IndexOptions=Index vector (dialog)  Indices=[4]  OutputSizes=1
  Selector{26..30} (5 alike) : Selector  InputPortWidth=12  IndexOptions=Index vector (dialog)  Indices=[10 11 12]  OutputSizes=1
  Selector{4..6,37..38} (5 alike) : Selector  InputPortWidth=12  IndexOptions=Index vector (dialog)  Indices=[1 2 3]  OutputSizes=1
  TIRE_MODE : ASM_VehicleDynamics_lib/VehicleDynamics/Tire/Common/TIRE_MODE  Tag=ASM_SUBCOMPONENT  ModeLeft=MDL.VehicleDynamics.Tire.ModeLeft  ModeRight=MDL.VehicleDynamics.Tire.ModeRight  ASMProperties=struct('Name','TIRE_MODE','Version','1.0','Library','ASM_VehicleDynamics_lib')  ASMInstanceName=tire_mode  ASMInstanceID=1
  Tire_FL : Subsystem
  Tire_FR : Subsystem
  Tire_RL : Subsystem
  Tire_RR : Subsystem
  p[Pa] : Constant  Value=220000
  ASMSignalBus : Outport
  F_Tire_CoorSys_V[FL,FR,RL,RR][x;y;z][N] : Outport  Port=2
  Trq_Tire_CoorSys_V[FL,FR,RL,RR][x;y;z][Nm] : Outport  Port=3
  Stiffness_z_Tire[FL,FR,RL,RR][N|m] : Outport  Port=4
  Trq_Tire_Wheel[FL,FR,RL,RR][Nm] : Outport  Port=5
  wires:
  TIRE_MODE/1 -> Demux/1
  Demux/2 -> Tire_FR/13(Mode[1Normal|2Mirror]), Tire_RR/13(Mode[1Normal|2Mirror])
  p[Pa]/1 -> Tire_FL/14(p[Pa]), Tire_RL/14(p[Pa]), Tire_RR/14(p[Pa]), Tire_FR/14(p[Pa])
  Demux/1 -> Tire_RL/13(Mode[1Normal|2Mirror]), Tire_FL/13(Mode[1Normal|2Mirror])
  Sat_TireParSet/1 -> Selector34/1, Selector33/1, Selector32/1, Selector31/1
  Sat_TireModel/1 -> Tire_FR/11(Sw_Tire_Model[1TMEasy|2MF]), Tire_RL/11(Sw_Tire_Model[1TMEasy|2MF]), Tire_RR/11(Sw_Tire_Model[1TMEasy|2MF]), ASMSignalCollector/1(Sw_Tire_Model), Tire_FL/11(Sw_Tire_Model[1TMEasy|2MF])
  Reset[]/1 -> Tire_FR/12(Reset[]), Tire_RL/12(Reset[]), Tire_RR/12(Reset[]), Tire_FL/12(Reset[])
  Mux5/1 -> Stiffness_z_Tire[FL,FR,RL,RR][N|m]/1
  Tire_RR/4(Stiffness_z_Tire[N|m]) -> Mux5/4
  Tire_RL/4(Stiffness_z_Tire[N|m]) -> Mux5/3
  Tire_FR/4(Stiffness_z_Tire[N|m]) -> Mux5/2
  Tire_FL/4(Stiffness_z_Tire[N|m]) -> Mux5/1
  [TAG_Sw_Tire_Model] -> Sat_TireModel/1
  Selector23/1 -> Tire_RR/1(Coeff_Fric_Road[])
  Selector25/1 -> Tire_RR/2(" Pos_z_CP_CoorSys_E[m]")
  Selector26/1 -> Tire_RR/3(UnitVec_z_CP_CoorSys_E[x;y;z])
  Selector27/1 -> Tire_RR/4(Pos_Wheels_CoorSys_E[x;y;z][m])
  Selector28/1 -> Tire_RR/5(v_WheelBody_Abs_CoorSys_V[x;y;z][m|s])
  Selector29/1 -> Tire_RR/6(w_Wheel_CoorSys_Abs_V[x;y;z][rad|s])
  Selector24/1 -> Tire_RR/9(omega_Wheel[rad|s])
  Selector30/1 -> Tire_RR/8(UnitVec_y_Wheel_CoorSys_V[x;y;z])
  Selector34/1 -> Tire_RR/10(Sw_Tire_Parameter_Set[1|2|3|4])
  Selector33/1 -> Tire_RL/10(Sw_Tire_Parameter_Set[1|2|3|4])
  Selector32/1 -> Tire_FR/10(Sw_Tire_Parameter_Set[1|2|3|4])
  Selector31/1 -> Tire_FL/10(Sw_Tire_Parameter_Set[1|2|3|4])
  Sw_Tire_Parameter_Set[FL,FR,RL,RR][1|2|3|4]/1 -> Sat_TireParSet/1
  Tire_RR/3(Trq_Tire_Wheel[Nm]) -> Mux3/4
  Tire_RL/3(Trq_Tire_Wheel[Nm]) -> Mux3/3
  Tire_FR/3(Trq_Tire_Wheel[Nm]) -> Mux3/2
  Tire_FL/3(Trq_Tire_Wheel[Nm]) -> Mux3/1
  Mux3/1 -> Trq_Tire_Wheel[FL,FR,RL,RR][Nm]/1
  Tire_RR/2(Trq_Tire[x;y;z][Nm]) -> Mux1/4
  Tire_RL/2(Trq_Tire[x;y;z][Nm]) -> Mux1/3
  Tire_FR/2(Trq_Tire[x;y;z][Nm]) -> Mux1/2
  Tire_FL/2(Trq_Tire[x;y;z][Nm]) -> Mux1/1
  Tire_RR/1(F_Tire[x;y;z][N]) -> Mux4/4
  Tire_RL/1(F_Tire[x;y;z][N]) -> Mux4/3
  Tire_FR/1(F_Tire[x;y;z][N]) -> Mux4/2
  Tire_FL/1(F_Tire[x;y;z][N]) -> Mux4/1
  Selector22/1 -> Tire_RL/9(omega_Wheel[rad|s])
  Selector21/1 -> Tire_RL/8(UnitVec_y_Wheel_CoorSys_V[x;y;z])
  Selector20/1 -> Tire_RL/6(w_Wheel_CoorSys_Abs_V[x;y;z][rad|s])
  Selector19/1 -> Tire_RL/5(v_WheelBody_Abs_CoorSys_V[x;y;z][m|s])
  Selector18/1 -> Tire_RL/4(Pos_Wheels_CoorSys_E[x;y;z][m])
  Selector17/1 -> Tire_RL/3(UnitVec_z_CP_CoorSys_E[x;y;z])
  Selector16/1 -> Tire_RL/2(" Pos_z_CP_CoorSys_E[m]")
  Selector15/1 -> Tire_RL/1(Coeff_Fric_Road[])
  Selector1/1 -> Tire_FR/9(omega_Wheel[rad|s])
  Selector7/1 -> Tire_FR/8(UnitVec_y_Wheel_CoorSys_V[x;y;z])
  Selector13/1 -> Tire_FR/6(w_Wheel_CoorSys_Abs_V[x;y;z][rad|s])
  Selector8/1 -> Tire_FR/5(v_WheelBody_Abs_CoorSys_V[x;y;z][m|s])
  Selector12/1 -> Tire_FR/4(Pos_Wheels_CoorSys_E[x;y;z][m])
  Selector11/1 -> Tire_FR/3(UnitVec_z_CP_CoorSys_E[x;y;z])
  Selector2/1 -> Tire_FR/2(" Pos_z_CP_CoorSys_E[m]")
  Selector14/1 -> Tire_FR/1(Coeff_Fric_Road[])
  Selector38/1 -> Tire_FL/6(w_Abs_Wheel_CoorSys_V[x;y;z][rad|s])
  w_Abs_Wheel_CoorSys_V[FL,FR,RL,RR][x,y,z][rad|s]/1 -> Selector29/1, Selector20/1, Selector13/1, Selector38/1
  Selector6/1 -> Tire_FL/5(v_Abs_WheelBody_CoorSys_V[x;y;z][m|s])
  v_Abs_WheelBody_CoorSys_V[FL,FR,RL,RR][x;y;z][m|s]/1 -> Selector28/1, Selector19/1, Selector8/1, Selector6/1
  Selector5/1 -> Tire_FL/4(Pos_Wheels_CoorSys_E[x;y;z][m])
  Pos_Wheels_CoorSys_E[FL,FR,RL,RR][x,y,z][m]/1 -> Selector27/1, Selector18/1, Selector12/1, Selector5/1
  Selector4/1 -> Tire_FL/3(UnitVec_z_CP_CoorSys_E[x;y;z])
  Coef_Fric_Road[FL,FR,RL,RR][]/1 -> Selector23/1, Selector15/1, Selector14/1, Selector9/1
  Selector9/1 -> Tire_FL/1(Coeff_Fric_Road[])
  Selector3/1 -> Tire_FL/2(" Pos_z_CP_CoorSys_E[m]")
  " Pos_z_CP_CoorSys_E[FL,FR,RL,RR][m]"/1 -> Selector3/1, Selector2/1, Selector25/1, Selector16/1
  UnitVec_z_CP_CoorSys_E[FL,FR,RL,RR][x;y;z]/1 -> Selector26/1, Selector17/1, Selector11/1, Selector4/1
  RotationMatrix_V_to_E_T[3x3]/1 -> Tire_FR/7(RotationMatrix_V_E_T[3x3]), Tire_RL/7(RotationMatrix_V_E_T[3x3]), Tire_RR/7(RotationMatrix_V_E_T[3x3]), Tire_FL/7(RotationMatrix_V_to_E_T[3x3])
  UnitVec_y_Wheel_CoorSys_V[FL,FR,RL,RR][x y z]/1 -> Selector30/1, Selector21/1, Selector7/1, Selector37/1
  Selector37/1 -> Tire_FL/8(UnitVec_y_Wheel_CoorSys_V[x;y;z])
  omega_Wheel[FL,FR,RL,RR][rad|s]/1 -> Selector24/1, Selector22/1, Selector1/1, Selector10/1
  Selector10/1 -> Tire_FL/9(omega_Wheel[rad|s])
  Mux1/1 -> Trq_Tire_CoorSys_V[FL,FR,RL,RR][x;y;z][Nm]/1
  Mux4/1 -> F_Tire_CoorSys_V[FL,FR,RL,RR][x;y;z][N]/1
  ASMSignalCollector/1(ASMSignalBus) -> ASMSignalBus/1

== system ASM_Traffic_V2X_Complete_Model_2/MDL/VehicleDynamics/VehicleInits ==
  q_dt_Vehicle_Init[6x1] : Inport
  Bus Selector : BusSelector  OutputSignals=Tire_FL.ActiveTire.r_Dyn_FL_Tire[m],Tire_FR.ActiveTire.r_Dyn_FR_Tire[m],Tire_RL.ActiveTire.r_Dyn_RL_Tire[m],Tire_RR.ActiveTire.r_Dyn_RR_Tire[m]
  Bus Selector1 : BusSelector  OutputSignals=q_dt_Wheel_Init[:],q_Wheel_Init[:]
  Mux : Mux  Inputs=2
  Mux1 : Mux
  Product : Product  Inputs=/*  RndMeth=Zero
  Saturation : Saturate  UpperLimit=inf  LowerLimit=0.01
  Unit Delay1 : UnitDelay  SampleTime=-1
  v_x_Init[m|s] : Selector  InputPortWidth=6  IndexOptions=Index vector (dialog)  Indices=[1]  OutputSizes=1
  omega_Wheel_Init[:][rad|s] : Outport
  q_dt_Init[:] : Outport  Port=2
  q_Wheel_Init[:] : Outport  Port=3
  wires:
  [ASMBUS_VehicleDynamics_Tire] -> Bus Selector/1
  Product/1 -> Unit Delay1/1
  Unit Delay1/1 -> omega_Wheel_Init[:][rad|s]/1
  Bus Selector/1 -> Mux1/1  "<r_Dyn_FL_Tire[m]>"
  Saturation/1 -> Product/1
  [TAG_Suspension_Init] -> Bus Selector1/1
  Bus Selector1/1 -> Mux/2  "<q_dt_Wheel_Init[:]>"
  Bus Selector1/2 -> q_Wheel_Init[:]/1  "<q_Wheel_Init[:]>"
  Mux/1 -> q_dt_Init[:]/1
  v_x_Init[m|s]/1 -> Product/2
  Bus Selector/2 -> Mux1/2  "<r_Dyn_FR_Tire[m]>"
  Bus Selector/3 -> Mux1/3  "<r_Dyn_RL_Tire[m]>"
  Bus Selector/4 -> Mux1/4  "<r_Dyn_RR_Tire[m]>"
  Mux1/1 -> Saturation/1
  q_dt_Vehicle_Init[6x1]/1 -> Mux/1, v_x_Init[m|s]/1
